simulink model "LAB1_3_real"  (R2025b)
settings: Solver=ode3  StartTime=0.0  StopTime=10  FixedStep=0.001  RelTol=1e-3
undefined symbols (not defined in the file or in its folder): degs2rpm, delta_c, den_Hi, den_Hw, K_g, KI, mot, National_Instruments, Nu, num_Hi, num_Hw, Nx, PCI, rpm2rads, sens, w_c
libraries: sldrtlib x3
settings Model: SimulationMode=external  ExtModeTrigDuration=100001  Creator=delpratogi  LastModifiedBy=Simone
settings DataIOCC: ReturnWorkspaceOutputs=off
settings HardwareCC: ProdBitPerLong=64.0  ProdHWDeviceType=Intel->x86-64 (Linux 64)
settings RTWCC: SystemTargetFile=sldrt.tlc  TemplateMakefile=sldrt.tmf  RTWCompilerOptimization=on  Description=Simulink Desktop Real-Time
settings CodeAppCC: MaxIdLength=95.0
settings STFCustomTargetCC: SystemTargetFile=sldrt.tlc  TargetLangStandard=C99 (ISO)  ModelReferenceCompliant=off  ConcurrentExecutionCompliant=off  MATLABClassNameForMDSCustomization=Simulink.SoftwareTarget.TargetSpecificTriggerConfigurationBase

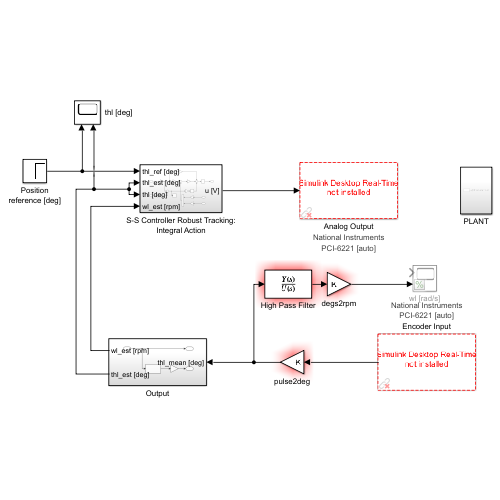
[thumbnail: Simulink's stored preview of the top-level diagram]
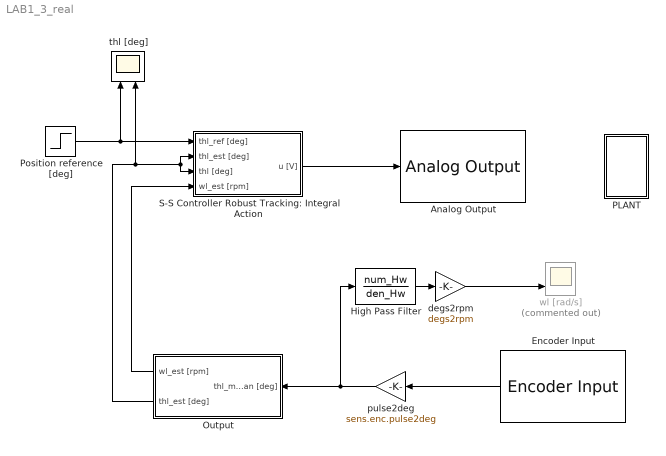
== system LAB1_3_real ==
  Analog Output : sldrtlib/Analog Output  SampleTime=0.001  MaxMissedTicks=10  ShowMissedTicks=off  YieldWhenWaiting=off  DrvName=National_Instruments/PCI-6221  DrvAddress=4294967295  DrvOptions=[0 0 0 2 0]  Channels=1  RangeMode=1  VoltRange=1  InitialValue=0  FinalValue=0
      settings: AttributesFormatString=National Instruments\nPCI-6221 [auto]
  Encoder Input : sldrtlib/Encoder Input  SampleTime=0.001  MaxMissedTicks=10  ShowMissedTicks=off  YieldWhenWaiting=off  DrvName=National_Instruments/PCI-6221  DrvAddress=4294967295  DrvOptions=[0 0 0 2 0]  Channels=1  QuadMode=3  IndexPulse=1  InputFilter=Inf  DataType=1
      settings: AttributesFormatString=National Instruments\nPCI-6221 [auto]
  High Pass Filter : TransferFcn  Numerator=num_Hw  Denominator=den_Hw
  Output : Subsystem
  PLANT : Subsystem
  Position reference [deg] : Step  Time=0  After=120  SampleTime=0  ZeroCross=off
  S-S Controller Robust Tracking: Integral Action : Subsystem
  degs2rpm : Gain  Gain=degs2rpm
  pulse2deg : Gain  Gain=sens.enc.pulse2deg
  thl [deg] : Scope  NumInputPorts=2
      settings: ActiveDisplayYMinimum=-21.42  ActiveDisplayYMaximum=192.78
  wl [rad/s] : Scope  Commented=on  NumInputPorts=2
      settings: ActiveDisplayYMinimum=345.16519  ActiveDisplayYMaximum=479.74204  DataLoggingVariableName=wl
  wires:
  Encoder Input/1 -> pulse2deg/1
  degs2rpm/1 -> wl [rad/s]/2
  High Pass Filter/1 -> degs2rpm/1
  pulse2deg/1 -> Output/1(thl_mean [deg]), High Pass Filter/1
  S-S Controller Robust Tracking: Integral Action/1(u [V]) -> Analog Output/1
  Output/1(wl_est [rpm]) -> S-S Controller Robust Tracking: Integral Action/4(wl_est [rpm])
  Position reference [deg]/1 -> S-S Controller Robust Tracking: Integral Action/1(thl_ref [deg]), thl [deg]/1
  Output/2(thl_est [deg]) -> thl [deg]/2, S-S Controller Robust Tracking: Integral Action/2(thl_est [deg]), S-S Controller Robust Tracking: Integral Action/3(thl [deg])

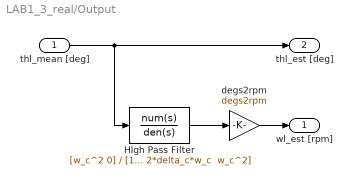
== system LAB1_3_real/Output ==
  thl_mean [deg] : Inport
  HIgh Pass Filter : TransferFcn  Numerator=[w_c^2 0]  Denominator="[1 2*delta_c*w_c  w_c^2]"
  degs2rpm : Gain  Gain=degs2rpm
  wl_est [rpm] : Outport
  thl_est [deg] : Outport  Port=2
  wires:
  thl_mean [deg]/1 -> HIgh Pass Filter/1, thl_est [deg]/1
  HIgh Pass Filter/1 -> degs2rpm/1
  degs2rpm/1 -> wl_est [rpm]/1

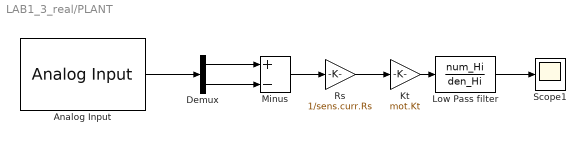
== system LAB1_3_real/PLANT ==
  Analog Input : sldrtlib/Analog Input  SampleTime=0.001  MaxMissedTicks=10  ShowMissedTicks=off  YieldWhenWaiting=off  DrvName=National_Instruments/PCI-6221  DrvAddress=4294967295  DrvOptions=[0 0 0 2 0]  Channels=[1,2]  RangeMode=1  VoltRange=1  DataType=1
      settings: AttributesFormatString=National Instruments\nPCI-6221 [auto]
  Demux : Demux  Outputs=2
  Kt : Gain  Gain=mot.Kt
  Low Pass filter : TransferFcn  Numerator=num_Hi  Denominator=den_Hi
  Minus : Sum  Inputs=+-
  Rs : Gain  Gain=1/sens.curr.Rs
  Scope1 : Scope
  wires:
  Low Pass filter/1 -> Scope1/1
  Demux/1 -> Minus/1
  Minus/1 -> Rs/1
  Analog Input/1 -> Demux/1
  Kt/1 -> Low Pass filter/1
  Demux/2 -> Minus/2
  Rs/1 -> Kt/1

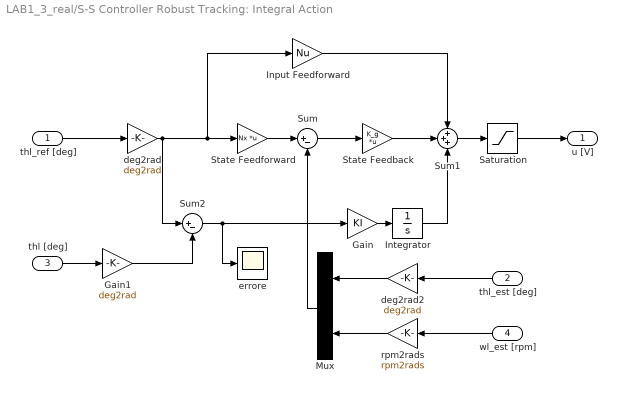
== system LAB1_3_real/S-S Controller Robust Tracking: Integral Action ==
  thl_ref [deg] : Inport
  thl_est [deg] : Inport  Port=2
  thl [deg] : Inport  Port=3
  wl_est [rpm] : Inport  Port=4
  Gain : Gain  Gain=KI
  Gain1 : Gain  Gain=deg2rad
  Input Feedforward : Gain  Gain=Nu
  Integrator : Integrator
  Mux : Mux  Inputs=2
  Saturation : Saturate  UpperLimit=10  LowerLimit=-10  ZeroCross=off
  State Feedback : Gain  Gain=K_g  Multiplication=Matrix(K*u)
  State Feedforward : Gain  Gain=Nx  Multiplication=Matrix(K*u)
  Sum : Sum  Inputs=|+-
  Sum1 : Sum  Inputs=+++
  Sum2 : Sum  Inputs=|+-
  deg2rad : Gain  Gain=deg2rad
  deg2rad2 : Gain  Gain=deg2rad
  errore : Scope
      settings: ActiveDisplayYMinimum=-1.27025  ActiveDisplayYMaximum=2.46824  DataLoggingVariableName=ScopeData2
  rpm2rads : Gain  Gain=rpm2rads
  u [V] : Outport
  wires:
  Saturation/1 -> u [V]/1
  wl_est [rpm]/1 -> rpm2rads/1
  thl_ref [deg]/1 -> deg2rad/1
  Sum1/1 -> Saturation/1
  deg2rad/1 -> Sum2/1, Input Feedforward/1, State Feedforward/1
  Mux/1 -> Sum/2
  Input Feedforward/1 -> Sum1/1
  Sum/1 -> State Feedback/1
  State Feedforward/1 -> Sum/1
  rpm2rads/1 -> Mux/2
  thl_est [deg]/1 -> deg2rad2/1
  deg2rad2/1 -> Mux/1
  State Feedback/1 -> Sum1/2
  Gain/1 -> Integrator/1
  Integrator/1 -> Sum1/3
  thl [deg]/1 -> Gain1/1
  Gain1/1 -> Sum2/2
  Sum2/1 -> errore/1, Gain/1
